simulink model "Resynchronization_Harness"  (R2025b)
settings: Solver=FixedStepAuto  StartTime=0.0  StopTime=10  RelTol=1e-3
PostLoadFcn:
  | ResynchronizationParam;
values from neighbouring files (symbols this model uses):
  Ts = 5E-5    (= 5e-05)    [BESSGFLParam.m]    (also in BESSGFMParam.m; WindFarmParam.m)
undefined symbols (not defined in the file or in its folder): resync
libraries: slpidlib x3, eeGeneralControl x3
settings Model: Creator=skota  LastModifiedBy=skota

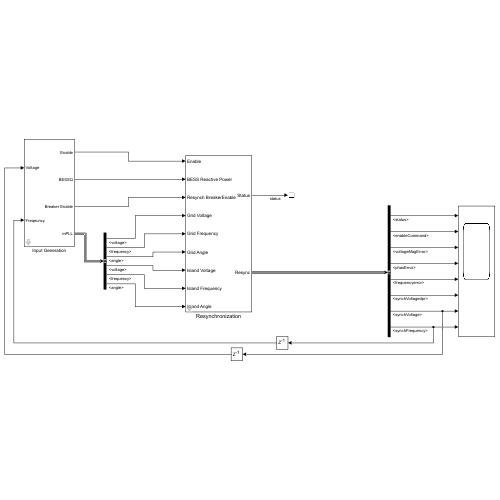
[thumbnail: Simulink's stored preview of the top-level diagram]
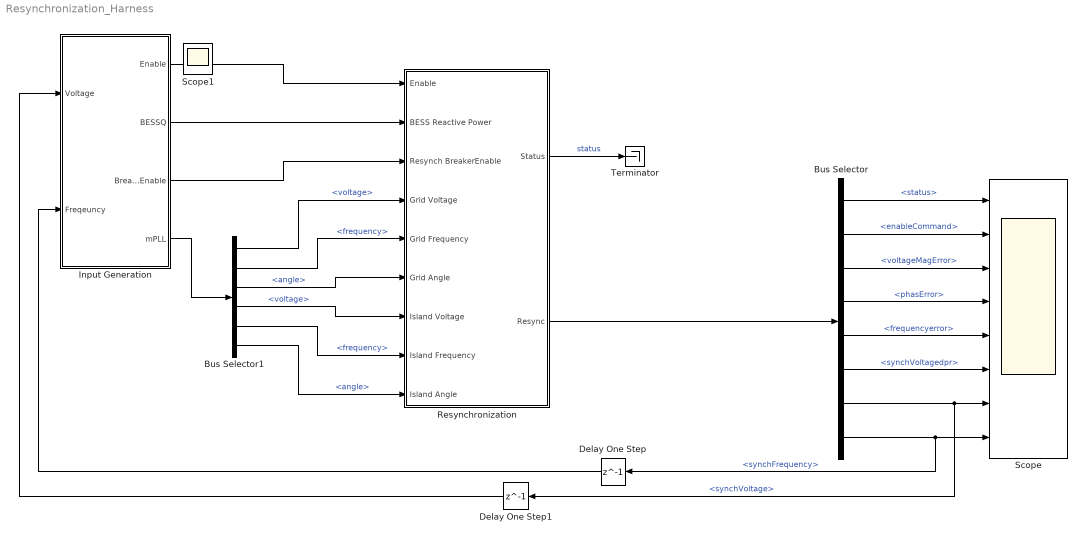
== system Resynchronization_Harness ==
  Bus Selector : BusSelector  OutputSignals=status,enableCommand,voltageMagError,phasError,frequencyerror,synchVoltagedpr,synchVoltage,synchFrequency
  Bus Selector1 : BusSelector  OutputSignals=Grid.voltage,Grid.frequency,Grid.angle,Island.voltage,Island.frequency,Island.angle
  Delay One Step : Delay  DelayLength=1
  Delay One Step1 : Delay  DelayLength=1
  Input Generation : Subsystem  mask{V=1, f=resync.gridFrequency, enCmdstart=2, enCmdstop=12, Q_BESS=0.5, resyncBreakTime=18}
      mask prompts: V "Voltage"; f "Frequency"; enCmdstart "EnableStart"; enCmdstop "EnableStop"; Q_BESS "BESS Reactive Power"; resyncBreakTime "ResyncBreak"
  Resynchronization : Subsystem  mask(Resynchronization){GridFrequency=resync.gridFrequency, KpVolResynch=resync.kpVoltage, KiVolResynch=resync.kiVoltage, VoltageThreshold=resync.vThreshold, kDroop=resync.vDroop, KpFreResynch=resync.kpFrequency, KiFreResynch=resync.kpFrequency, FrequencyThreshold=resync.fThreshold, KpAngResynch=resync.kpAngle, KiAngResynch=resync.kiAngle, AngleThreshold=resync.aThreshold}
      mask prompts: GridFrequency "Grid Frequency"; KpVolResynch "Proportional Gain"; KiVolResynch "Integral Gain"; kDroop "Voltage Droop"; KpFreResynch "Proportional Gain"; KiFreResynch "Integral Gain"; KpAngResynch "Proportional Gain"; KiAngResynch "Integral Gain"
      mask help: This block enables the microgrid to reconnect with the grid if the voltage, frequency and angle of the islanded microgrid matches to the grid with certain threshold
      settings: CopyFcn=set_param(gcbh,'LinkStatus','none');
      mask Help: web('Resynchronization.html')
      mask DialogControl Container4 Prompt: General
      mask DialogControl Container6 Prompt: Voltage
      mask DialogControl Container5 Prompt: Frequency
      mask DialogControl Container7 Prompt: Angle
  Scope : Scope  NumInputPorts=8
      settings: ActiveDisplayYMinimum=-0.12499999999999997  ActiveDisplayYMaximum=1.125
  Terminator : Terminator
  Scope1 : Scope
      settings: DataLoggingVariableName=ScopeData3
  wires:
  Resynchronization/2(Resync) -> Bus Selector/1
  Resynchronization/1(Status) -> Terminator/1  "status"
  Bus Selector/1 -> Scope/1  "<status>"
  Bus Selector/2 -> Scope/2  "<enableCommand>"
  Bus Selector/3 -> Scope/3  "<voltageMagError>"
  Bus Selector/4 -> Scope/4  "<phasError>"
  Bus Selector/5 -> Scope/5  "<frequencyerror>"
  Bus Selector/6 -> Scope/6  "<synchVoltagedpr>"
  Bus Selector/7 -> Delay One Step1/1, Scope/7  "<synchVoltage>"
  Bus Selector/8 -> Delay One Step/1, Scope/8  "<synchFrequency>"
  Input Generation/2(BESSQ) -> Resynchronization/2(BESS Reactive Power)
  Delay One Step/1 -> Input Generation/2(Freqeuncy)
  Delay One Step1/1 -> Input Generation/1(Voltage)
  Bus Selector1/6 -> Resynchronization/9(Island Angle)  "<angle>"
  Input Generation/3(Breaker Enable) -> Resynchronization/3(Resynch BreakerEnable)
  Input Generation/4(mPLL) -> Bus Selector1/1
  Bus Selector1/1 -> Resynchronization/4(Grid Voltage)  "<voltage>"
  Bus Selector1/2 -> Resynchronization/5(Grid Frequency)  "<frequency>"
  Bus Selector1/3 -> Resynchronization/6(Grid Angle)  "<angle>"
  Bus Selector1/4 -> Resynchronization/7(Island Voltage)  "<voltage>"
  Bus Selector1/5 -> Resynchronization/8(Island Frequency)  "<frequency>"
  Input Generation/1(Enable) -> Resynchronization/1(Enable)

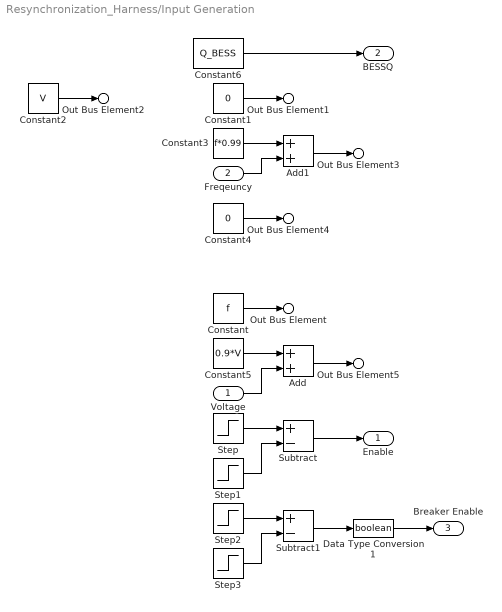
== system Resynchronization_Harness/Input Generation ==
  Voltage : Inport
  Freqeuncy : Inport  Port=2
  Add : Sum
  Add1 : Sum
  Constant : Constant  Value=f
  Constant1 : Constant  Value=0
  Constant2 : Constant  Value=V
  Constant3 : Constant  Value=f*0.99
  Constant4 : Constant  Value=0
  Constant5 : Constant  Value=0.9*V
  Constant6 : Constant  Value=Q_BESS
  Data Type Conversion1 : DataTypeConversion  OutDataTypeStr=boolean  SaturateOnIntegerOverflow=off  RndMeth=Floor
  Step : Step  Time=enCmdstart  SampleTime=0
  Step1 : Step  Time=enCmdstop  SampleTime=0
  Step2 : Step  Time=resyncBreakTime  SampleTime=0
  Step3 : Step  Time=resyncBreakTime+2  SampleTime=0
  Subtract : Sum  Inputs=+-
  Subtract1 : Sum  Inputs=+-
  Enable : Outport  OutDataTypeStr=double
  BESSQ : Outport  Port=2
  Breaker Enable : Outport  Port=3
  Out Bus Element2 : Outport  Port=4  PortName=mPLL  Element=Grid.voltage
  Out Bus Element : Outport  Port=4  PortName=mPLL  Element=Grid.frequency
  Out Bus Element1 : Outport  Port=4  PortName=mPLL  Element=Grid.angle
  Out Bus Element5 : Outport  Port=4  PortName=mPLL  Element=Island.voltage
  Out Bus Element3 : Outport  Port=4  PortName=mPLL  Element=Island.frequency
  Out Bus Element4 : Outport  Port=4  PortName=mPLL  Element=Island.angle
  wires:
  Add/1 -> Out Bus Element5/1
  Voltage/1 -> Add/2
  Constant6/1 -> BESSQ/1
  Constant1/1 -> Out Bus Element1/1
  Constant/1 -> Out Bus Element/1
  Constant3/1 -> Add1/1
  Constant2/1 -> Out Bus Element2/1
  Freqeuncy/1 -> Add1/2
  Constant5/1 -> Add/1
  Step/1 -> Subtract/1
  Step1/1 -> Subtract/2
  Step2/1 -> Subtract1/1
  Step3/1 -> Subtract1/2
  Add1/1 -> Out Bus Element3/1
  Data Type Conversion1/1 -> Breaker Enable/1
  Subtract1/1 -> Data Type Conversion1/1
  Subtract/1 -> Enable/1
  Constant4/1 -> Out Bus Element4/1

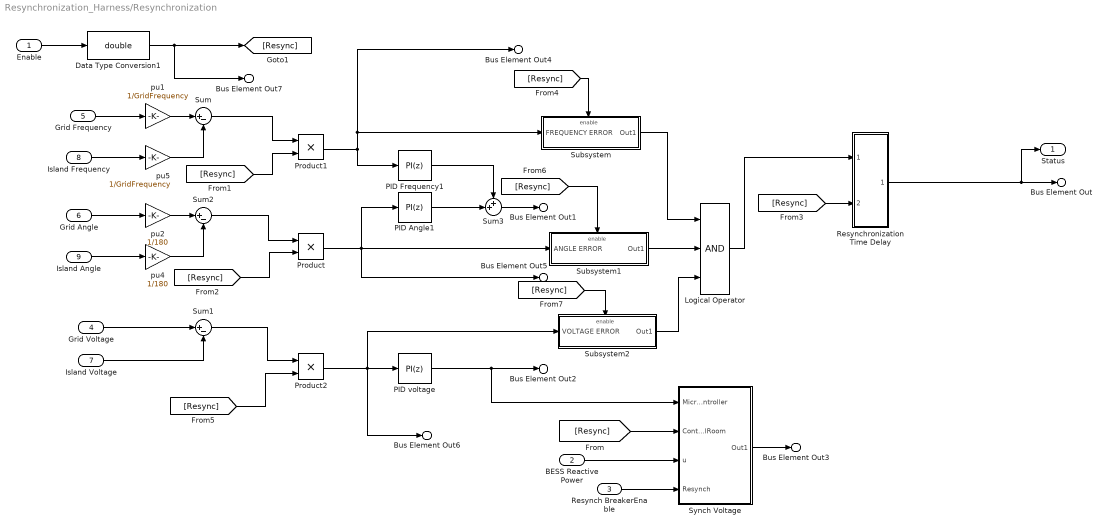
== system Resynchronization_Harness/Resynchronization ==
  Enable : Inport
  BESS Reactive Power : Inport  Port=2
  Resynch BreakerEnable : Inport  Port=3
  Grid Voltage : Inport  Port=4
  Grid Frequency : Inport  Port=5
  Grid Angle : Inport  Port=6
  Island Voltage : Inport  Port=7
  Island Frequency : Inport  Port=8
  Island Angle : Inport  Port=9
  Data Type Conversion1 : DataTypeConversion  OutDataTypeStr=double  SaturateOnIntegerOverflow=off  RndMeth=Floor
  Logical Operator : Logic  Inputs=3  AllPortsSameDT=off  OutDataTypeStr=boolean
  PID Angle1 : slpidlib/PID Controller  Controller=PI  Form=Parallel  TimeDomain=Discrete-time  UseExternalTs=off  SampleTime=Ts  IntegratorMethod=Forward Euler  FilterMethod=Forward Euler  ControllerParametersSource=internal  P=KpAngResynch  I=KiAngResynch  UseKiTs=off  D=0  UseExternalDerivativeSource=off  N=100  UseFilter=on  TunerSelectOption=Frequency Response Based  InitialConditionSource=internal  InitialConditionForIntegrator=0  InitialConditionForFilter=0  DifferentiatorICPrevScaledInput=0  ExternalReset=none  TrackingMode=off  Kt=1  LimitOutput=off  SatLimitsSource=internal  UpperSaturationLimit=0.5  LowerSaturationLimit=-0.5  LinearizeAsGain=on  AntiWindupMode=clamping  Kb=1  LimitIntegrator=off  UpperIntegratorSaturationLimit=inf  LowerIntegratorSaturationLimit=-inf  POutMin=[]  POutMax=[]  IOutMin=[]  IOutMax=[]  DOutMin=[]  DOutMax=[]  NOutMin=[]  NOutMax=[]  SumOutMin=[]  SumOutMax=[]  SaturationOutMin=[]  SaturationOutMax=[]  PParamMin=[]  PParamMax=[]  IParamMin=[]  IParamMax=[]  DParamMin=[]  DParamMax=[]  NParamMin=[]  NParamMax=[]  KbParamMin=[]  KbParamMax=[]  KtParamMin=[]  KtParamMax=[]  KbOutMin=[]  KbOutMax=[]  KtOutMin=[]  KtOutMax=[]  IntegratorOutMin=[]  IntegratorOutMax=[]  FilterOutMin=[]  FilterOutMax=[]  SumI1OutMin=[]  SumI1OutMax=[]  SumI2OutMin=[]  SumI2OutMax=[]  SumI3OutMin=[]  SumI3OutMax=[]  SumI4OutMin=[]  SumI4OutMax=[]  SumDOutMin=[]  SumDOutMax=[]  DifferentiatorOutMin=[]  DifferentiatorOutMax=[]  FilterDiffOutCoefMin=[]  FilterDiffOutCoefMax=[]  ReciprocalOutMin=[]  ReciprocalOutMax=[]  SumDenOutMin=[]  SumDenOutMax=[]  SumNumOutMin=[]  SumNumOutMax=[]  DivideOutMin=[]  DivideOutMax=[]  UdiffTsProdOutMin=[]  UdiffTsProdOutMax=[]  NTsProdOutMin=[]  NTsProdOutMax=[]  UintegralTsProdOutMin=[]  UintegralTsProdOutMax=[]  UngainTsProdOutMin=[]  UngainTsProdOutMax=[]  ClampingZeroOutDataTypeStr=Inherit: Inherit via back propagation  ClampingZeroOutMin=[]  ClampingZeroOutMax=[]  FilterDenConstantOutDataTypeStr=Inherit: Inherit via back propagation  FilterDenConstantOutMin=[]  FilterDenConstantOutMax=[]  PCopyOutDataTypeStr=Inherit: Inherit via back propagation  PCopyOutMin=[]  PCopyOutMax=[]  NCopyOutDataTypeStr=Inherit: Inherit via back propagation  NCopyOutMin=[]  NCopyOutMax=[]  IntegratorContinuousStateAttributes=''  IntegratorStateMustResolveToSignalObject=off  IntegratorRTWStateStorageClass=Auto  FilterContinuousStateAttributes=''  FilterStateMustResolveToSignalObject=off  FilterRTWStateStorageClass=Auto  ParallelPVariant=InternalParameters  IdealPVariant=Disabled  IVariant=InternalParameters  DVariant=Disabled  IntegratorVariant=Discrete  SatVariant=Disabled  AWVariant=Passthrough  PCopyVariant=Disabled  TRVariant=Disabled  FdbkBlocksVariant=Forward  IdealPFdbkVariant=Disabled  SatFdbkVariant=Disabled  DerivativeFilterVariant=Disabled  NVariant=Disabled  NCopyVariant=Disabled_SignalSpec  FilterICVariant=Disabled  IntegratorICVariant=InternalICs  ExternalResetVariant=Disabled  TRSumVariant=Passthrough  SumFdbkVariant=Disabled  SumVariant=Sum_PI  TsampFilterVariant=InternalTs  TsampNgainVariant=Passthrough  TsampIntegralVariant=Disabled_SignalSpec  ExternalSaturationOutDataTypeStr=Inherit: Same as second input  DerivativeSourceVariant=Disabled  PreIntVariant=InternalPreInt
  PID Frequency1 : slpidlib/PID Controller  Controller=PI  Form=Parallel  TimeDomain=Discrete-time  UseExternalTs=off  SampleTime=Ts  IntegratorMethod=Forward Euler  FilterMethod=Forward Euler  ControllerParametersSource=internal  P=KpFreResynch  I=KiFreResynch  UseKiTs=off  D=0  UseExternalDerivativeSource=off  N=100  UseFilter=on  TunerSelectOption=Frequency Response Based  InitialConditionSource=internal  InitialConditionForIntegrator=0  InitialConditionForFilter=0  DifferentiatorICPrevScaledInput=0  ExternalReset=none  TrackingMode=off  Kt=1  LimitOutput=off  SatLimitsSource=internal  UpperSaturationLimit=0.05  LowerSaturationLimit=-0.05  LinearizeAsGain=on  AntiWindupMode=clamping  Kb=1  LimitIntegrator=off  UpperIntegratorSaturationLimit=inf  LowerIntegratorSaturationLimit=-inf  POutMin=[]  POutMax=[]  IOutMin=[]  IOutMax=[]  DOutMin=[]  DOutMax=[]  NOutMin=[]  NOutMax=[]  SumOutMin=[]  SumOutMax=[]  SaturationOutMin=[]  SaturationOutMax=[]  PParamMin=[]  PParamMax=[]  IParamMin=[]  IParamMax=[]  DParamMin=[]  DParamMax=[]  NParamMin=[]  NParamMax=[]  KbParamMin=[]  KbParamMax=[]  KtParamMin=[]  KtParamMax=[]  KbOutMin=[]  KbOutMax=[]  KtOutMin=[]  KtOutMax=[]  IntegratorOutMin=[]  IntegratorOutMax=[]  FilterOutMin=[]  FilterOutMax=[]  SumI1OutMin=[]  SumI1OutMax=[]  SumI2OutMin=[]  SumI2OutMax=[]  SumI3OutMin=[]  SumI3OutMax=[]  SumI4OutMin=[]  SumI4OutMax=[]  SumDOutMin=[]  SumDOutMax=[]  DifferentiatorOutMin=[]  DifferentiatorOutMax=[]  FilterDiffOutCoefMin=[]  FilterDiffOutCoefMax=[]  ReciprocalOutMin=[]  ReciprocalOutMax=[]  SumDenOutMin=[]  SumDenOutMax=[]  SumNumOutMin=[]  SumNumOutMax=[]  DivideOutMin=[]  DivideOutMax=[]  UdiffTsProdOutMin=[]  UdiffTsProdOutMax=[]  NTsProdOutMin=[]  NTsProdOutMax=[]  UintegralTsProdOutMin=[]  UintegralTsProdOutMax=[]  UngainTsProdOutMin=[]  UngainTsProdOutMax=[]  ClampingZeroOutDataTypeStr=Inherit: Inherit via back propagation  ClampingZeroOutMin=[]  ClampingZeroOutMax=[]  FilterDenConstantOutDataTypeStr=Inherit: Inherit via back propagation  FilterDenConstantOutMin=[]  FilterDenConstantOutMax=[]  PCopyOutDataTypeStr=Inherit: Inherit via back propagation  PCopyOutMin=[]  PCopyOutMax=[]  NCopyOutDataTypeStr=Inherit: Inherit via back propagation  NCopyOutMin=[]  NCopyOutMax=[]  IntegratorContinuousStateAttributes=''  IntegratorStateMustResolveToSignalObject=off  IntegratorRTWStateStorageClass=Auto  FilterContinuousStateAttributes=''  FilterStateMustResolveToSignalObject=off  FilterRTWStateStorageClass=Auto  ParallelPVariant=InternalParameters  IdealPVariant=Disabled  IVariant=InternalParameters  DVariant=Disabled  IntegratorVariant=Discrete  SatVariant=Disabled  AWVariant=Passthrough  PCopyVariant=Disabled  TRVariant=Disabled  FdbkBlocksVariant=Forward  IdealPFdbkVariant=Disabled  SatFdbkVariant=Disabled  DerivativeFilterVariant=Disabled  NVariant=Disabled  NCopyVariant=Disabled_SignalSpec  FilterICVariant=Disabled  IntegratorICVariant=InternalICs  ExternalResetVariant=Disabled  TRSumVariant=Passthrough  SumFdbkVariant=Disabled  SumVariant=Sum_PI  TsampFilterVariant=InternalTs  TsampNgainVariant=Passthrough  TsampIntegralVariant=Disabled_SignalSpec  ExternalSaturationOutDataTypeStr=Inherit: Same as second input  DerivativeSourceVariant=Disabled  PreIntVariant=InternalPreInt
  PID voltage : slpidlib/PID Controller  Controller=PI  Form=Parallel  TimeDomain=Discrete-time  UseExternalTs=off  SampleTime=Ts  IntegratorMethod=Forward Euler  FilterMethod=Forward Euler  ControllerParametersSource=internal  P=KpVolResynch  I=KiVolResynch  UseKiTs=off  D=0  UseExternalDerivativeSource=off  N=100  UseFilter=on  TunerSelectOption=Frequency Response Based  InitialConditionSource=internal  InitialConditionForIntegrator=1  InitialConditionForFilter=0  DifferentiatorICPrevScaledInput=0  ExternalReset=none  TrackingMode=off  Kt=1  LimitOutput=off  SatLimitsSource=internal  UpperSaturationLimit=1.5  LowerSaturationLimit=-0.05  LinearizeAsGain=on  AntiWindupMode=clamping  Kb=1  LimitIntegrator=off  UpperIntegratorSaturationLimit=inf  LowerIntegratorSaturationLimit=-inf  POutMin=[]  POutMax=[]  IOutMin=[]  IOutMax=[]  DOutMin=[]  DOutMax=[]  NOutMin=[]  NOutMax=[]  SumOutMin=[]  SumOutMax=[]  SaturationOutMin=[]  SaturationOutMax=[]  PParamMin=[]  PParamMax=[]  IParamMin=[]  IParamMax=[]  DParamMin=[]  DParamMax=[]  NParamMin=[]  NParamMax=[]  KbParamMin=[]  KbParamMax=[]  KtParamMin=[]  KtParamMax=[]  KbOutMin=[]  KbOutMax=[]  KtOutMin=[]  KtOutMax=[]  IntegratorOutMin=[]  IntegratorOutMax=[]  FilterOutMin=[]  FilterOutMax=[]  SumI1OutMin=[]  SumI1OutMax=[]  SumI2OutMin=[]  SumI2OutMax=[]  SumI3OutMin=[]  SumI3OutMax=[]  SumI4OutMin=[]  SumI4OutMax=[]  SumDOutMin=[]  SumDOutMax=[]  DifferentiatorOutMin=[]  DifferentiatorOutMax=[]  FilterDiffOutCoefMin=[]  FilterDiffOutCoefMax=[]  ReciprocalOutMin=[]  ReciprocalOutMax=[]  SumDenOutMin=[]  SumDenOutMax=[]  SumNumOutMin=[]  SumNumOutMax=[]  DivideOutMin=[]  DivideOutMax=[]  UdiffTsProdOutMin=[]  UdiffTsProdOutMax=[]  NTsProdOutMin=[]  NTsProdOutMax=[]  UintegralTsProdOutMin=[]  UintegralTsProdOutMax=[]  UngainTsProdOutMin=[]  UngainTsProdOutMax=[]  ClampingZeroOutDataTypeStr=Inherit: Inherit via back propagation  ClampingZeroOutMin=[]  ClampingZeroOutMax=[]  FilterDenConstantOutDataTypeStr=Inherit: Inherit via back propagation  FilterDenConstantOutMin=[]  FilterDenConstantOutMax=[]  PCopyOutDataTypeStr=Inherit: Inherit via back propagation  PCopyOutMin=[]  PCopyOutMax=[]  NCopyOutDataTypeStr=Inherit: Inherit via back propagation  NCopyOutMin=[]  NCopyOutMax=[]  IntegratorContinuousStateAttributes=''  IntegratorStateMustResolveToSignalObject=off  IntegratorRTWStateStorageClass=Auto  FilterContinuousStateAttributes=''  FilterStateMustResolveToSignalObject=off  FilterRTWStateStorageClass=Auto  ParallelPVariant=InternalParameters  IdealPVariant=Disabled  IVariant=InternalParameters  DVariant=Disabled  IntegratorVariant=Discrete  SatVariant=Disabled  AWVariant=Passthrough  PCopyVariant=Disabled  TRVariant=Disabled  FdbkBlocksVariant=Forward  IdealPFdbkVariant=Disabled  SatFdbkVariant=Disabled  DerivativeFilterVariant=Disabled  NVariant=Disabled  NCopyVariant=Disabled_SignalSpec  FilterICVariant=Disabled  IntegratorICVariant=InternalICs  ExternalResetVariant=Disabled  TRSumVariant=Passthrough  SumFdbkVariant=Disabled  SumVariant=Sum_PI  TsampFilterVariant=InternalTs  TsampNgainVariant=Passthrough  TsampIntegralVariant=Disabled_SignalSpec  ExternalSaturationOutDataTypeStr=Inherit: Same as second input  DerivativeSourceVariant=Disabled  PreIntVariant=InternalPreInt
  Product : Product
  Product1 : Product
  Product2 : Product
  Resynchronization Time Delay : Subsystem
  Subsystem : Subsystem
  Subsystem1 : Subsystem
  Subsystem2 : Subsystem
  Sum : Sum  Inputs=|+-
  Sum1 : Sum  Inputs=|+-
  Sum2 : Sum  Inputs=|+-
  Sum3 : Sum  Inputs=++|
  Synch Voltage : Subsystem
  pu1 : Gain  Gain=1/GridFrequency
  pu2 : Gain  Gain=1/180
  pu4 : Gain  Gain=1/180
  pu5 : Gain  Gain=1/GridFrequency
  Status : Outport
  Bus Element Out : Outport  Port=2  PortName=Resync  Element=status
  Bus Element Out1 : Outport  Port=2  PortName=Resync  Element=synchFrequency
  Bus Element Out2 : Outport  Port=2  PortName=Resync  Element=synchVoltage
  Bus Element Out3 : Outport  Port=2  PortName=Resync  Element=synchVoltagedpr
  Bus Element Out4 : Outport  Port=2  PortName=Resync  Element=frequencyerror
  Bus Element Out5 : Outport  Port=2  PortName=Resync  Element=phasError
  Bus Element Out6 : Outport  Port=2  PortName=Resync  Element=voltageMagError
  Bus Element Out7 : Outport  Port=2  PortName=Resync  Element=enableCommand
  wires:
  PID Frequency1/1 -> Sum3/1
  pu1/1 -> Sum/1
  Resynch BreakerEnable/1 -> Synch Voltage/4(Resynch)
  Island Voltage/1 -> Sum1/2
  Product1/1 -> Bus Element Out4/1, Subsystem/1(FREQUENCY ERROR), PID Frequency1/1
  Sum2/1 -> Product/1
  pu4/1 -> Sum2/2
  BESS Reactive Power/1 -> Synch Voltage/3(u)
  PID Angle1/1 -> Sum3/2
  Island Frequency/1 -> pu5/1
  pu2/1 -> Sum2/1
  Data Type Conversion1/1 -> Bus Element Out7/1, [Resync]
  Product2/1 -> PID voltage/1, Bus Element Out6/1, Subsystem2/1(VOLTAGE ERROR)
  Grid Voltage/1 -> Sum1/1
  Island Angle/1 -> pu4/1
  [Resync] -> Product1/2
  Grid Angle/1 -> pu2/1
  Grid Frequency/1 -> pu1/1
  Product/1 -> Bus Element Out5/1, Subsystem1/1(ANGLE ERROR), PID Angle1/1
  Subsystem/1(Out1) -> Logical Operator/1
  Resynchronization Time Delay/1(MGController) -> Bus Element Out/1, Status/1
  pu5/1 -> Sum/2
  [Resync] -> Product2/2
  [Resync] -> Resynchronization Time Delay/2(In2)
  Logical Operator/1 -> Resynchronization Time Delay/1(In1)
  [Resync] -> Synch Voltage/2(ControlRoom)
  Subsystem2/1(Out1) -> Logical Operator/3
  Subsystem1/1(Out1) -> Logical Operator/2
  [Resync] -> Subsystem2/Enable
  Synch Voltage/1(Out1) -> Bus Element Out3/1
  Sum1/1 -> Product2/1
  Enable/1 -> Data Type Conversion1/1
  Sum3/1 -> Bus Element Out1/1
  Sum/1 -> Product1/1
  PID voltage/1 -> Bus Element Out2/1, Synch Voltage/1(MicrogridController)
  [Resync] -> Subsystem/Enable
  [Resync] -> Product/2
  [Resync] -> Subsystem1/Enable

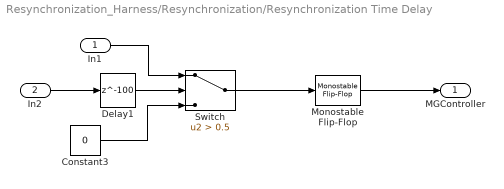
== system Resynchronization_Harness/Resynchronization/Resynchronization Time Delay ==
  In1 : Inport
  In2 : Inport  Port=2
  Constant3 : Constant  Value=0
  Delay1 : Delay  DelayLength=100  SampleTime=Ts
  Monostable Flip-Flop : eeGeneralControl/Monostable Flip-Flop  VariantControl=Variant1  LabelModeActiveChoice=Discrete  ChangeType=Rising edge  x0=0  Td=100  Ts=Ts
      settings: LibrarySourceBlock=ee_sl_lib/General Control/Monostable Flip-Flop
  Switch : Switch  Criteria=u2 > Threshold  Threshold=0.5  SaturateOnIntegerOverflow=off  InputSameDT=off
  MGController : Outport
  wires:
  In2/1 -> Delay1/1
  In1/1 -> Switch/1
  Monostable Flip-Flop/1 -> MGController/1
  Delay1/1 -> Switch/2
  Constant3/1 -> Switch/3
  Switch/1 -> Monostable Flip-Flop/1

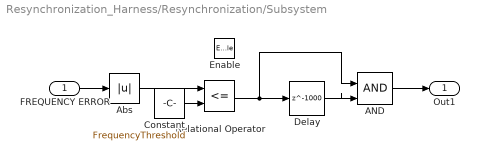
== system Resynchronization_Harness/Resynchronization/Subsystem ==
  FREQUENCY ERROR : Inport
  Enable : EnablePort
  AND : Logic  IconShape=distinctive  AllPortsSameDT=off  OutDataTypeStr=boolean
  Abs : Abs  SaturateOnIntegerOverflow=off
  Constant : Constant  Value=FrequencyThreshold  SampleTime=-1
  Delay : Delay  DelayLength=1000  SampleTime=Ts
  Relational Operator : RelationalOperator  Operator=<=  OutDataTypeStr=boolean  RndMeth=Simplest  InputSameDT=off
  Out1 : Outport
  wires:
  Abs/1 -> Relational Operator/1
  FREQUENCY ERROR/1 -> Abs/1
  AND/1 -> Out1/1
  Relational Operator/1 -> Delay/1, AND/1
  Constant/1 -> Relational Operator/2
  Delay/1 -> AND/2

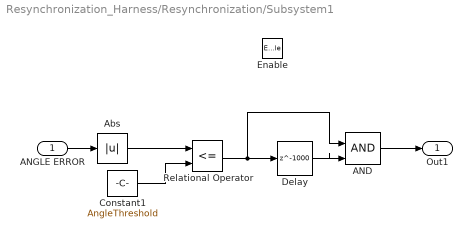
== system Resynchronization_Harness/Resynchronization/Subsystem1 ==
  ANGLE ERROR : Inport
  Enable : EnablePort
  AND : Logic  IconShape=distinctive  AllPortsSameDT=off  OutDataTypeStr=boolean
  Abs : Abs  SaturateOnIntegerOverflow=off
  Constant1 : Constant  Value=AngleThreshold
  Delay : Delay  DelayLength=1000  SampleTime=Ts
  Relational Operator : RelationalOperator  Operator=<=  OutDataTypeStr=boolean  RndMeth=Simplest  InputSameDT=off
  Out1 : Outport
  wires:
  Abs/1 -> Relational Operator/1
  Delay/1 -> AND/2
  Constant1/1 -> Relational Operator/2
  Relational Operator/1 -> AND/1, Delay/1
  AND/1 -> Out1/1
  ANGLE ERROR/1 -> Abs/1

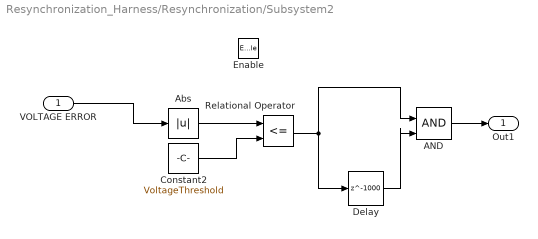
== system Resynchronization_Harness/Resynchronization/Subsystem2 ==
  VOLTAGE ERROR : Inport
  Enable : EnablePort
  AND : Logic  IconShape=distinctive  AllPortsSameDT=off  OutDataTypeStr=boolean
  Abs : Abs  SaturateOnIntegerOverflow=off
  Constant2 : Constant  Value=VoltageThreshold
  Delay : Delay  DelayLength=1000  SampleTime=Ts
  Relational Operator : RelationalOperator  Operator=<=  OutDataTypeStr=boolean  RndMeth=Simplest  InputSameDT=off
  Out1 : Outport
  wires:
  Abs/1 -> Relational Operator/1
  VOLTAGE ERROR/1 -> Abs/1
  AND/1 -> Out1/1
  Relational Operator/1 -> Delay/1, AND/1
  Constant2/1 -> Relational Operator/2
  Delay/1 -> AND/2

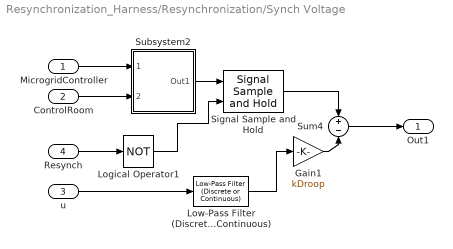
== system Resynchronization_Harness/Resynchronization/Synch Voltage ==
  MicrogridController : Inport
  ControlRoom : Inport  Port=2
  u : Inport  Port=3
  Resynch : Inport  Port=4
  Gain1 : Gain  Gain=kDroop
  Logical Operator1 : Logic  Operator=NOT  AllPortsSameDT=off  OutDataTypeStr=boolean
  Low-Pass Filter (Discrete or Continuous) : eeGeneralControl/Low-Pass Filter (Discrete or Continuous)  K=1  T=0.08  B=inf  A=-inf  init_option=Specify as parameter  x0=0  Ts=5*Ts
  Signal Sample and Hold : eeGeneralControl/Signal Sample and Hold  LabelModeActiveChoice=Discrete  x0=1  Ts=Ts
      settings: LibrarySourceBlock=ee_sl_lib/General Control/Signal Sample and Hold
  Subsystem2 : Subsystem
  Sum4 : Sum  Inputs=+-
  Out1 : Outport
  wires:
  u/1 -> Low-Pass Filter (Discrete or Continuous)/1
  ControlRoom/1 -> Subsystem2/2(ControlRoom)
  Sum4/1 -> Out1/1
  Subsystem2/1(Out1) -> Signal Sample and Hold/1
  MicrogridController/1 -> Subsystem2/1(MicrogridController)
  Logical Operator1/1 -> Signal Sample and Hold/2
  Gain1/1 -> Sum4/2
  Signal Sample and Hold/1 -> Sum4/1
  Resynch/1 -> Logical Operator1/1
  Low-Pass Filter (Discrete or Continuous)/1 -> Gain1/1

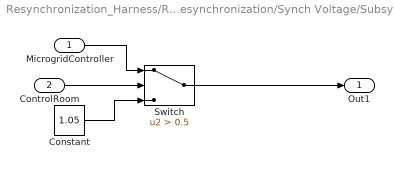
== system Resynchronization_Harness/Resynchronization/Synch Voltage/Subsystem2 ==
  MicrogridController : Inport
  ControlRoom : Inport  Port=2
  Constant : Constant  Value=1.05
  Switch : Switch  Criteria=u2 > Threshold  Threshold=0.5  SaturateOnIntegerOverflow=off  InputSameDT=off
  Out1 : Outport
  wires:
  MicrogridController/1 -> Switch/1
  ControlRoom/1 -> Switch/2
  Constant/1 -> Switch/3
  Switch/1 -> Out1/1
